simulink model "test_lift_motion_law"  (R2021b)
settings: Solver=VariableStepAuto  StartTime=0.0  StopTime=600  RelTol=1e-3
values from neighbouring files (symbols this model uses):
  floor_height = 3    [load_data.m]    (also in run_test_motion_logic.m; test_motion_law.m; test_switched.m)
  gearbox = 1    [load_data.m]    (also in run_test_motion_law_block.m; run_test_motion_logic.m; test_motion_law.m)
  Rp = 0.5    [load_data.m]    (also in run_test_motion_law_block.m; run_test_motion_logic.m; test_motion_law.m)
  Ts = 1e-3    (= 0.001)    [load_data.m]    (also in run_test_motion_law_block.m; run_test_motion_logic.m; run_test_switch_sensor.m; testWegMotionLaw.m)
libraries: LiftMotionControlLibrary x4, slpidlib x1
settings Model: Creator=manue  LastModifiedBy=manue
settings ConfigComp: PLC_TargetIDE=generic  PLC_MultiTBSigbuilderTimeRange=off  PLC_InlineEnumCastFunction=off

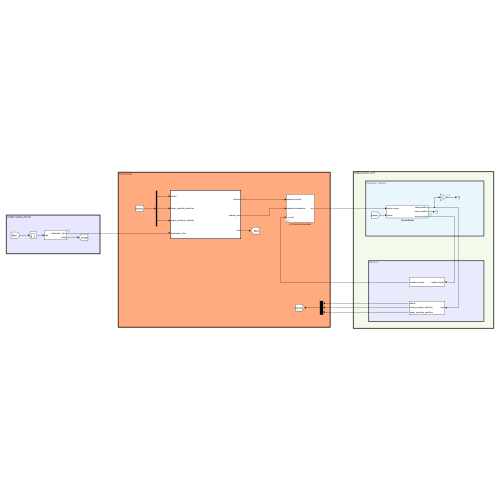
[thumbnail: Simulink's stored preview of the top-level diagram]
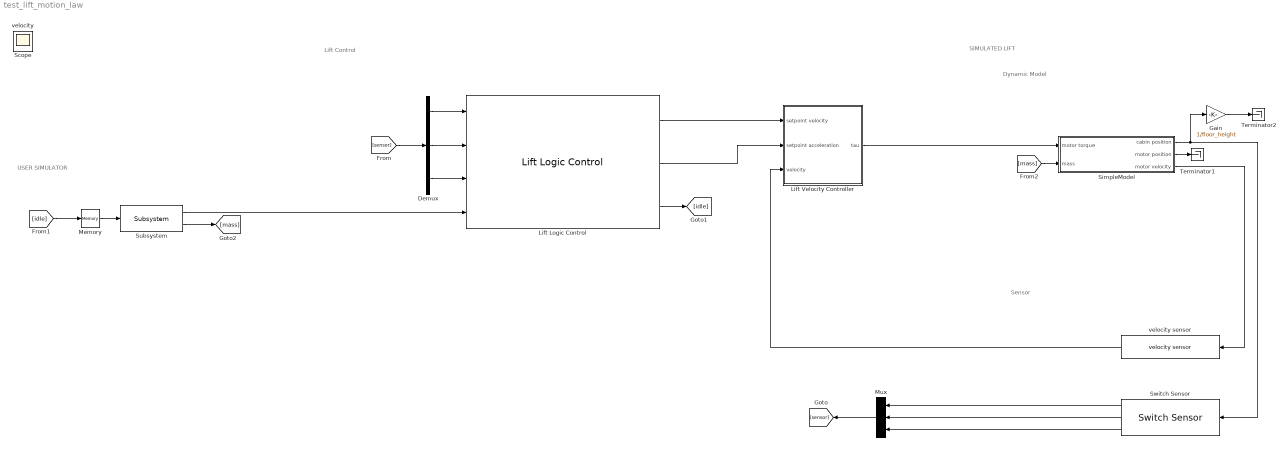
== system test_lift_motion_law ==
  note: SIMULATED LIFT
  note: USER SIMULATOR
  note: Sensor
  note: Dynamic Model
  note: Lift Control
  Demux : Demux  Outputs=3
  Gain : Gain  Gain=1/floor_height
  Lift Logic Control : LiftMotionControlLibrary/Lift Logic Control  floor_height=floor_height  num_floors=num_floors  cabin_height=cabin_height  proximity_distance=proximity_distance  waiting_time=waiting_time  MinVel=MinVel  MaxVel=MaxVel  Ts=Ts  MaxAcc=MaxAcc  MaxJerk=MaxJerk  gearbox=gearbox  cabin_offset=cabin_offset  Rp=Rp  motion_profile=Profile 1: single speed
  Lift Velocity Controller : Subsystem  AncestorBlock=LiftMotionControlLibrary/Lift Velocity Controller
  Memory : Memory
  Mux : Mux  Inputs=3
  SimpleModel : Subsystem
  Subsystem : LiftMotionControlLibrary/Subsystem  SystemSampleTime=-1  VariantActivationTime=update diagram  Latency=0  AutoFrameSizeCalculation=off
  Switch Sensor : LiftMotionControlLibrary/Switch Sensor  floor_height=floor_height  num_floors=num_floors  proximity_distance=proximity_distance  cabin_height=cabin_height
  Terminator1 : Terminator
  Terminator2 : Terminator
  velocity sensor : LiftMotionControlLibrary/velocity sensor  SystemSampleTime=-1  VariantActivationTime=update diagram  Latency=0  AutoFrameSizeCalculation=off
  Scope : Scope
  velocity : Scope
  wires:
  Subsystem/1 -> Lift Logic Control/4
  SimpleModel/1(cabin position) -> Gain/1, Switch Sensor/1
  Switch Sensor/1 -> Mux/1
  Switch Sensor/2 -> Mux/2
  Switch Sensor/3 -> Mux/3
  Demux/3 -> Lift Logic Control/3
  Demux/2 -> Lift Logic Control/2
  Demux/1 -> Lift Logic Control/1
  Mux/1 -> [sensor]
  [sensor] -> Demux/1
  SimpleModel/2(motor position) -> Terminator1/1
  Lift Logic Control/1 -> Lift Velocity Controller/1(setpoint velocity)
  velocity sensor/1 -> Lift Velocity Controller/3(velocity)
  Lift Velocity Controller/1(tau) -> SimpleModel/1(motor torque)
  Lift Logic Control/2 -> Lift Velocity Controller/2(setpoint acceleration)
  Lift Logic Control/3 -> [idle]
  Subsystem/2 -> [mass]
  [mass] -> SimpleModel/2(mass)
  [idle] -> Memory/1
  Memory/1 -> Subsystem/1
  SimpleModel/3(motor velocity) -> velocity sensor/1
  Gain/1 -> Terminator2/1

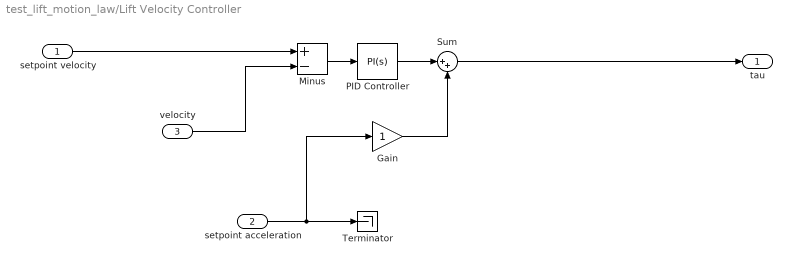
== system test_lift_motion_law/Lift Velocity Controller ==
  setpoint velocity : Inport
  setpoint acceleration : Inport  Port=2
  velocity : Inport  Port=3
  Gain : Gain
  Minus : Sum  Inputs=+-
  PID Controller : slpidlib/PID Controller  Controller=PI  Form=Parallel  TimeDomain=Continuous-time  UseExternalTs=off  SampleTime=-1  IntegratorMethod=Forward Euler  FilterMethod=Forward Euler  ControllerParametersSource=internal  P=50  I=5  D=0  UseFilter=on  N=100  TunerSelectOption=Transfer Function Based (PID Tuner App)  InitialConditionSource=internal  InitialConditionForIntegrator=0  InitialConditionForFilter=0  DifferentiatorICPrevScaledInput=0  ExternalReset=none  TrackingMode=off  Kt=1  LimitOutput=off  SatLimitsSource=internal  UpperSaturationLimit=inf  LowerSaturationLimit=-inf  LinearizeAsGain=on  AntiWindupMode=none  Kb=1  POutMin=[]  POutMax=[]  IOutMin=[]  IOutMax=[]  DOutMin=[]  DOutMax=[]  NOutMin=[]  NOutMax=[]  SumOutMin=[]  SumOutMax=[]  SaturationOutMin=[]  SaturationOutMax=[]  PParamMin=[]  PParamMax=[]  IParamMin=[]  IParamMax=[]  DParamMin=[]  DParamMax=[]  NParamMin=[]  NParamMax=[]  KbParamMin=[]  KbParamMax=[]  KtParamMin=[]  KtParamMax=[]  KbOutMin=[]  KbOutMax=[]  KtOutMin=[]  KtOutMax=[]  IntegratorOutMin=[]  IntegratorOutMax=[]  FilterOutMin=[]  FilterOutMax=[]  SumI1OutMin=[]  SumI1OutMax=[]  SumI2OutMin=[]  SumI2OutMax=[]  SumI3OutMin=[]  SumI3OutMax=[]  SumI4OutMin=[]  SumI4OutMax=[]  SumDOutMin=[]  SumDOutMax=[]  DifferentiatorOutMin=[]  DifferentiatorOutMax=[]  FilterDiffOutCoefMin=[]  FilterDiffOutCoefMax=[]  ReciprocalOutMin=[]  ReciprocalOutMax=[]  SumDenOutMin=[]  SumDenOutMax=[]  SumNumOutMin=[]  SumNumOutMax=[]  DivideOutMin=[]  DivideOutMax=[]  UdiffTsProdOutMin=[]  UdiffTsProdOutMax=[]  NTsProdOutMin=[]  NTsProdOutMax=[]  UintegralTsProdOutMin=[]  UintegralTsProdOutMax=[]  UngainTsProdOutMin=[]  UngainTsProdOutMax=[]  IntegratorContinuousStateAttributes=''  IntegratorStateMustResolveToSignalObject=off  IntegratorRTWStateStorageClass=Auto  FilterContinuousStateAttributes=''  FilterStateMustResolveToSignalObject=off  FilterRTWStateStorageClass=Auto  ParallelPVariant=InternalParameters  IdealPVariant=Disabled  IVariant=InternalParameters  DVariant=Disabled  IntegratorVariant=Continuous  SatVariant=Disabled  AWVariant=Passthrough  PCopyVariant=Disabled  TRVariant=Disabled  FdbkBlocksVariant=Forward  IdealPFdbkVariant=Disabled  SatFdbkVariant=Disabled  DerivativeFilterVariant=Disabled  NVariant=Disabled  NCopyVariant=Disabled_SignalSpec  FilterICVariant=Disabled  IntegratorICVariant=InternalICs  ExternalResetVariant=Disabled  TRSumVariant=Passthrough  SumFdbkVariant=Disabled  SumVariant=Sum_PI  TsampFilterVariant=InternalTs  TsampNgainVariant=Passthrough  TsampIntegralVariant=Passthrough  ExternalSaturationOutDataTypeStr=Inherit: Same as second input
  Sum : Sum  Inputs=|++
  Terminator : Terminator
  tau : Outport
  wires:
  Gain/1 -> Sum/2
  Sum/1 -> tau/1
  PID Controller/1 -> Sum/1
  setpoint velocity/1 -> Minus/1
  Minus/1 -> PID Controller/1
  velocity/1 -> Minus/2
  setpoint acceleration/1 -> Terminator/1, Gain/1

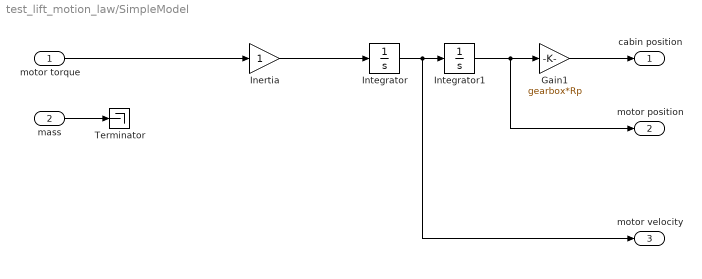
== system test_lift_motion_law/SimpleModel ==
  motor torque : Inport
  mass : Inport  Port=2
  Gain1 : Gain  Gain=gearbox*Rp
  Inertia : Gain
  Integrator : Integrator
  Integrator1 : Integrator
  Terminator : Terminator
  cabin position : Outport
  motor position : Outport  Port=2
  motor velocity : Outport  Port=3
  wires:
  Integrator/1 -> motor velocity/1, Integrator1/1
  Inertia/1 -> Integrator/1
  motor torque/1 -> Inertia/1
  Integrator1/1 -> motor position/1, Gain1/1
  Gain1/1 -> cabin position/1
  mass/1 -> Terminator/1
